simulink model "top_model"  (R2025a)
settings: Solver=ode45  StartTime=0.0  StopTime=2.5  RelTol=1e-3  EnableMultiTasking=on
libraries: spsSeriesRLCBranchLib x3, spsCurrentMeasurementLib x2, spsVoltageMeasurementLib x2, SignalEditorBlockLib x2, spsDiodeLib x1, spsIGBTLib x1, spsPVArrayLib x1, spsPWMGeneratorDCDCLib x1, spsSeriesRLCLoadLib x1, sps_lib x1
settings Model: Creator=The MathWorks, Inc.  LastModifiedBy=Asus
settings SolverCC: AlgebraicLoopSolver=TrustRegion
settings DataIOCC: LimitDataPoints=on  ReturnWorkspaceOutputs=off
settings OptimizationCC: LifeSpan=inf
settings DebuggingCC: UnconnectedInputMsg=warning  UnconnectedOutputMsg=warning  UnconnectedLineMsg=warning  AllowSymbolicDim=off  SFUnexpectedBacktrackingDiag=warning  SFNoUnconditionalDefaultTransitionDiag=warning  SFExecutionAtInitializationDiag=none  ArithmeticOperatorsInVariantConditions=warning
settings ModelReferenceCC: EnableRefExpFcnMdlSchedulingChecks=on  PropagateSignalLabelsOutOfModel=off
settings SFSimCC: SimUseLocalCustomCode=off  CustomCodeUndefinedFunction=UseInterfaceOnly
settings RTWCC: RTWUseLocalCustomCode=off  GPUComputeCapability=3.5
settings CodeAppCC: StateflowObjectComments=on
settings GRTTargetCC: TargetLangStandard=C89/C90 (ANSI)
settings ConfigComp: CovMetricSettings=dw  CovSaveCumulativeToWorkspaceVar=on  CovSaveSingleToWorkspaceVar=on  CovExternalEMLEnable=off

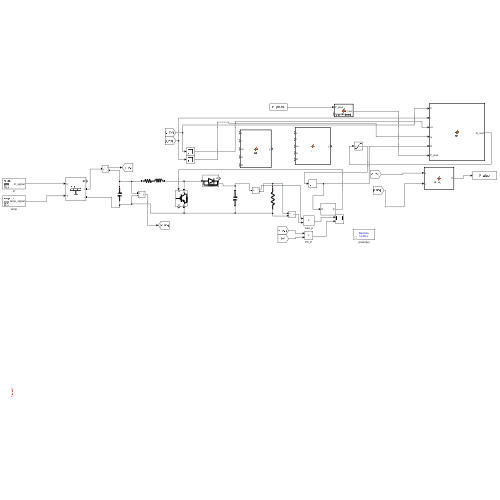
[thumbnail: Simulink's stored preview of the top-level diagram]
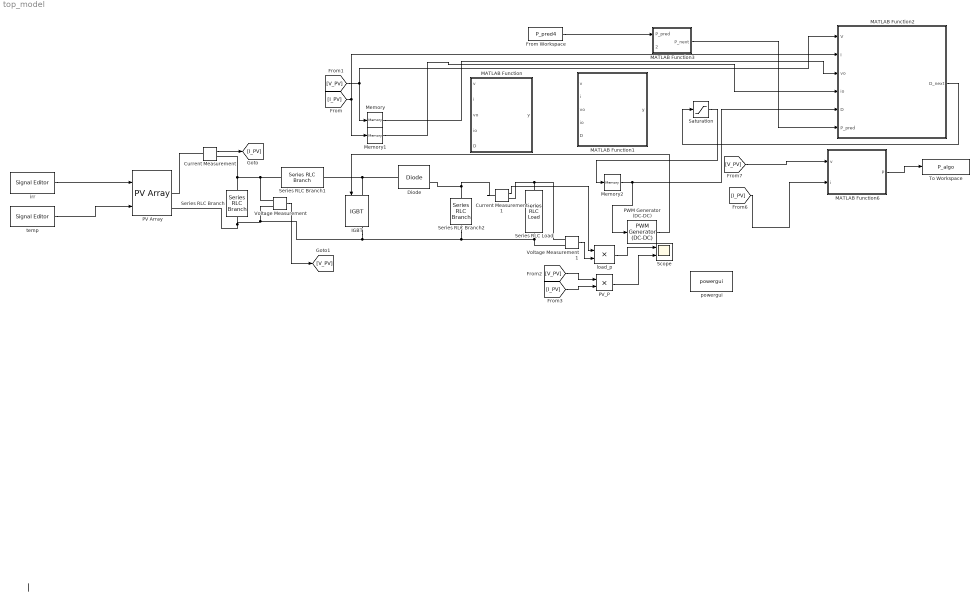
== system top_model ==
  Current Measurement : spsCurrentMeasurementLib/Current Measurement  PhasorSimulation=off  OutputType=Complex  PSBequivalent=0
  Current Measurement1 : spsCurrentMeasurementLib/Current Measurement  PhasorSimulation=off  OutputType=Complex  PSBequivalent=0
  Diode : spsDiodeLib/Diode  Ron=0.001  Lon=0  Vf=0.8  IC=0  UseSnubber=0  Rs=500  Cs=250e-9  Measurements=on
  From Workspace : FromWorkspace  VariableName=P_pred4  SampleTime=0.01
  IGBT : spsIGBTLib/IGBT  Ron=0.001  Lon=0  Vf=1  Tf=1e-6  Tt=2e-6  IC=0  Rs=1e5  Cs=inf  Measurements=on
  MATLAB Function : MATLAB Function  TreatAsAtomicUnit=on
  MATLAB Function1 : MATLAB Function  TreatAsAtomicUnit=on
  MATLAB Function2 : MATLAB Function  TreatAsAtomicUnit=on
  MATLAB Function3 : MATLAB Function  TreatAsAtomicUnit=on
  MATLAB Function6 : MATLAB Function  TreatAsAtomicUnit=on
  Memory : Memory
  Memory1 : Memory
  Memory2 : Memory
  PV Array : spsPVArrayLib/PV Array  Npar=66  Nser=10  PlotType=array @ 1000 W/m2 & specified temperatures  S_vec="[ 1000  500  100 ]"  Temp_C_vec="[ 45 25  ]"  ModuleName=User-defined  PlotWhenSelected=off  Pm=305.226  Ncell=96  Voc=64.2  Isc=5.96  Vm=54.7  Im=5.58  beta_Voc_pc=-0.177  alpha_Isc_pc=0.003516  beta_Voc=-0.11363  alpha_Isc=0.00020955  IL=5.9893  I0=3.2313e-14  nI=0.79323  Rsh=279.5394  Rs=0.53126  RobustModel=off  RobustCellTemperature=313.3991  BAL=on  Tc=1e-6  Tfilter=5e-5
  PV_P : Product
  PWM Generator (DC-DC) : spsPWMGeneratorDCDCLib/PWM Generator (DC-DC)  Fsw=5000  Ts=0
  Saturation : Saturate  UpperLimit=0.9  LowerLimit=0
  Scope : Scope  NumInputPorts=2
      settings: ActiveDisplayYMinimum=-0.098373784311174411  ActiveDisplayYMaximum=0.88536405880057
  Series RLC Branch : spsSeriesRLCBranchLib/Series RLC Branch  LConnTagsString=__new0  RConnTagsString=__new0  BranchType=C  Resistance=1  Inductance=1e-3  SetiL0=off  InitialCurrent=0  Capacitance=100e-6  Setx0=off  InitialVoltage=0  Measurements=None
  Series RLC Branch1 : spsSeriesRLCBranchLib/Series RLC Branch  LConnTagsString=__new0  RConnTagsString=__new0  BranchType=RL  Resistance=0.005  Inductance=0.005  SetiL0=off  InitialCurrent=0  Capacitance=1e-6  Setx0=off  InitialVoltage=0  Measurements=None
  Series RLC Branch2 : spsSeriesRLCBranchLib/Series RLC Branch  LConnTagsString=__new0  RConnTagsString=__new0  BranchType=C  Resistance=1  Inductance=1e-3  SetiL0=off  InitialCurrent=0  Capacitance=12000e-6  Setx0=off  InitialVoltage=0  Measurements=None
  Series RLC Load : spsSeriesRLCLoadLib/Series RLC Load  LConnTagsString=a  RConnTagsString=__new0  NominalVoltage=500  NominalFrequency=50  ActivePower=100e3  InductivePower=0  CapacitivePower=0  Setx0=off  InitialVoltage=0  SetiL0=off  InitialCurrent=0  Measurements=None  LoadType=constant Z
  To Workspace : ToWorkspace  VariableName=P_algo  SaveFormat=Timeseries  SampleTime=-1
  Voltage Measurement : spsVoltageMeasurementLib/Voltage Measurement  PhasorSimulation=off  OutputType=Complex  PSBequivalent=0
  Voltage Measurement1 : spsVoltageMeasurementLib/Voltage Measurement  PhasorSimulation=off  OutputType=Complex  PSBequivalent=0
  irr : SignalEditorBlockLib/Signal Editor  FileName=irr_dataset3.mat  ActiveScenario=irr_ds  ActiveSignal=irr_signal  IsBus=off  OutputBusObjectStr=Bus: BusObject  SampleTime=0.01  ZeroCross=off  OutputAfterFinalValue=Setting to zero  Unit=inherit  PreserveSignalName=on  ApplySigPropsToAllScenarios=off  ApplySigPropsToAllSignals=off  SignalPropertySource=Dialog parameters
  load_p : Product
  powergui : sps_lib/powergui  Priority=1  SimulationMode=Discrete  SampleTime=1e-06  frequency=60  Iterations=50  frequencyindice=0  Pbase=100e6  ErrMax=1e-4  UnitsV=kV  UnitsW=MW  buscounter=0  FunctionMessages=off  echomessages=off  EnableUseOfTLC=off  CurrentSourceSwitches=off  DisableSnubberDevices=off  DisableRonSwitches=off  DisableVfSwitches=off  DisplayEquations=off  AutomaticDiscreteSolvers=off  SolverType=Tustin/Backward Euler (TBE)  Interpol=off  ExternalGateDelay=off  methode=off  Ts=100  x0status=blocks  SPID=on  SwTol=0  HookPort=off  NonlinearTolerance=1e-4  nMaxIteration=100  ContinueOnMaxIteration=off  RestoreLinks=warning  ResistiveCurrentMeasurement=off  Frange=[0:2:500]  Ylog=off  Xlog=on  ShowGrid=off  save=off  variable=ZData  structure=0  ZoomFFT=off  StartTime=0.0  cycles=1  DisplayStyle=1  fundamental=60  FreqAxis=off  MaxFrequency=1000  frequencyindicesteady=1  RmsSteady=1  display=off
  temp : SignalEditorBlockLib/Signal Editor  FileName=temp_dataset3.mat  ActiveScenario=temp_ds  ActiveSignal=temp_signal  IsBus=off  OutputBusObjectStr=Bus: BusObject  SampleTime=0.01  ZeroCross=off  OutputAfterFinalValue=Setting to zero  Unit=inherit  PreserveSignalName=on  ApplySigPropsToAllScenarios=on  ApplySigPropsToAllSignals=off  SignalPropertySource=Dialog parameters
  wires:
  irr/1 -> PV Array/1
  temp/1 -> PV Array/2
  Current Measurement/1 -> [I_PV]
  Voltage Measurement/1 -> [V_PV]
  [V_PV] -> MATLAB Function2/1(V), Memory/1
  [I_PV] -> MATLAB Function2/2(I), Memory1/1
  Saturation/1 -> Memory2/1
  Memory2/1 -> MATLAB Function2/5(D), PWM Generator (DC-DC)/1
  PWM Generator (DC-DC)/1 -> IGBT/1
  Current Measurement1/1 -> load_p/1
  Voltage Measurement1/1 -> load_p/2
  load_p/1 -> Scope/1
  [V_PV] -> PV_P/1
  [I_PV] -> PV_P/2
  PV_P/1 -> Scope/2
  Memory/1 -> MATLAB Function2/3(vo)
  Memory1/1 -> MATLAB Function2/4(io)
  From Workspace/1 -> MATLAB Function3/1(P_pred)
  MATLAB Function3/1(P_next) -> MATLAB Function2/6(P_pred)
  MATLAB Function6/1(P) -> To Workspace/1
  [V_PV] -> MATLAB Function6/1(v)
  [I_PV] -> MATLAB Function6/2(i)
  MATLAB Function2/1(D_next) -> Saturation/1
  connections:
  Current Measurement/LConn1 -- PV Array/RConn1
  Series RLC Branch/RConn1 -- Voltage Measurement1/LConn2 -- Series RLC Load/RConn1 -- Series RLC Branch2/RConn1 -- IGBT/RConn1 -- Voltage Measurement/LConn2 -- PV Array/RConn2
  Voltage Measurement/LConn1 -- Series RLC Branch1/LConn1 -- Series RLC Branch/LConn1 -- Current Measurement/RConn1
  IGBT/LConn1 -- Diode/LConn1 -- Series RLC Branch1/RConn1
  Series RLC Branch2/LConn1 -- Current Measurement1/LConn1 -- Diode/RConn1
  Voltage Measurement1/LConn1 -- Current Measurement1/RConn1 -- Series RLC Load/LConn1
  ?

== matlab function top_model/MATLAB Function1 ==
  data: v input; y output; i input; vo input; io input; D input
function y = po(v, i, vo, io, D)
% MPPT Perturb & Observe (P&O)

d = 5e-5;      % step size
eps = 1e-6;    % small tolerance

% Power
P  = v  * i;
Po = vo * io;

% Delta
dP = P - Po;
dV = v - vo;

m = D;

if abs(dP) < eps
    % Power not change -> keep duty
    m = D;
else
    if dP > 0
        % Power increased
        if dV > 0
            m = D + d;
        else
            m = D - d;
        end
    else
        % Power decreased
        if dV > 0
            m = D - d;
        else
            m = D + d;
        end
    end
end

% Limit duty cycle
m = min(max(m, 0), 1);

y = m;
end

== matlab function top_model/MATLAB Function ==
  data: v input; y output; i input; vo input; io input; D input
function y = inc(v, i, vo, io, D)

d = 5e-5;
eps = 1e-6;

dv = v - vo;
di = i - io;

m = D;

if abs(dv) < eps
    if abs(di) < eps
        m = D;
    elseif di > 0
        m = D - d;
    else
        m = D + d;
    end
else
    if abs(di/dv + i/v) < eps
        m = D;
    elseif di/dv > -i/v
        m = D - d;
    else
        m = D + d;
    end
end

% limit duty cycle
m = min(max(m,0),1);

y = m;
end

== matlab function top_model/MATLAB Function2 ==
  data: V input; D_next output; I input; vo input; io input; D input; P_pred input
function D_next = fcn(V,I,vo,io,D,P_pred)
%#codegen
% AI-MPPT with Temporal Fusion (PAST + FUTURE)
% Codegen & Simulink safe implementation

%% ===== Persistent States =====
persistent init V_f I_f P_hist V_hist ai_conf momentum converge_cnt pred_mom

if isempty(init)
    init = true;
    V_f = V;
    I_f = I;

    P_hist = ones(10,1)*(V*I);
    V_hist = ones(10,1)*V;

    ai_conf = 0.8;
    momentum = 0;
    converge_cnt = 0;
    pred_mom = 0;
end

%% ===== Constants =====
Vmpp_stc = 54.7;
Pmpp_stc = Vmpp_stc*5.58;

D_min = 0.05;
D_max = 0.95;

d_min = 1.5e-4;
d_max = 0.02;

alpha_v = 0.82;
ai_thr  = 0.30;
ai_decay = 0.96;
err_gain = 10;

mom_k = 0.55;
rate_n = 0.05;
rate_f = 0.10;

%% ===== Input Protection =====
if vo == 0, vo = V; end
if io == 0, io = I; end

%% ===== Adaptive Filtering =====
is_tr = (abs(V-vo) > 0.5) || (abs(I-io) > 0.1);
if is_tr
    a = 0.68;
else
    a = alpha_v;
end

V_f = a*V + (1-a)*V_f;
I_f = a*I + (1-a)*I_f;
P_now = V_f*I_f;

%% ===== Update History =====
P_hist(1:end-1) = P_hist(2:end);
P_hist(end) = P_now;

V_hist(1:end-1) = V_hist(2:end);
V_hist(end) = V_f;

P_diff = diff(P_hist);     % 9x1
V_diff = diff(V_hist);     % 9x1

%% ===== PAST: Trend & Gradient =====
weights = [0.03;0.05;0.07;0.10;0.13;0.15;0.17;0.20;0.10];
trend_score = sum(weights .* sign(P_diff));

% Gradient estimation (safe)
sum_g = 0;
cnt_g = 0;
for k = 1:9
    if abs(V_diff(k)) > 1e-3
        sum_g = sum_g + P_diff(k)/V_diff(k);
        cnt_g = cnt_g + 1;
    end
end

if cnt_g > 0
    avg_gradient = sum_g/cnt_g;
    gradient_stable = true;
else
    avg_gradient = 0;
    gradient_stable = false;
end

%% ===== Consistency =====
consistency = 0;
for k = 6:9
    if sign(P_diff(k)) == sign(P_diff(9))
        consistency = consistency + 1;
    end
end
consistency = consistency / 4;

%% ===== FUTURE: AI Prediction =====
P_pred_ok = (P_pred > 1) && (P_pred < 2*Pmpp_stc);

if P_pred_ok
    P_err = (P_pred - P_now)/max(P_pred,1);
    qual = 1 - min(abs(P_err),1);
    ai_conf = 0.35*qual + 0.65*ai_conf;

    pred_dir = sign(P_pred - P_now);
    pred_mom = 0.7*pred_mom + 0.3*pred_dir;

    gain = 0.18 + 0.12*min(abs(P_err),0.6);
    Vmpp_pred = V_f + gain*Vmpp_stc*sign(P_err);
else
    P_err = 0;
    ai_conf = max(ai_conf*ai_decay,0.3);
    Vmpp_pred = V_f;
end

%% ===== FUSION =====
if ai_conf > 0.7 && P_pred_ok
    w_p = 0.3; w_f = 0.7;
elseif ai_conf > 0.5 && P_pred_ok
    w_p = 0.5; w_f = 0.5;
else
    w_p = 0.7; w_f = 0.3;
end

if abs(avg_gradient) > 0.1
    dir_past = sign(avg_gradient);
else
    dir_past = sign(trend_score);
end
if dir_past == 0, dir_past = 1; end

dir_future = sign(Vmpp_pred - V_f);
dir = sign(w_p*dir_past + w_f*dir_future);
if dir == 0, dir = 1; end
if P_pred_ok && abs(P_err) < 0.03
    dir = sign(dir + 0.35*sign(P_pred - P_now));
end
if dir == 0
    dir = 1;
end

%% ===== Convergence =====
near_pred = abs(P_err) < 0.012;
near_grad = gradient_stable && abs(avg_gradient) < 0.5;

if near_pred && near_grad
    converge_cnt = min(converge_cnt+1,20);
else
    converge_cnt = max(converge_cnt-1,0);
end
converged = (converge_cnt > 12) && (abs(avg_gradient) < 0.3);


%% ===== Step Size =====
if ai_conf > ai_thr && P_pred_ok
    mag = min(abs(P_err)*err_gain,1);
    step = d_min + (d_max-d_min)*mag;
else
    step = d_min*2;
end

if consistency > 0.7
    step = step*1.2;
end

step = min(step,d_max);

%% ===== Momentum =====
momentum = mom_k*momentum + (1-mom_k)*step;

if converged
    step_f = max(momentum*0.30, d_min*3);
elseif near_pred
    step_f = momentum*0.45;
else
    step_f = momentum;
end


%% ===== Duty Update =====
D_raw = D + dir*step_f;

Vmpp_hat = w_p*V_f + w_f*Vmpp_pred;
D_phy_max = min(D_max, max(1 - Vmpp_hat/max(V_f,1), D_min));

D_next = min(max(D_raw,D_min),D_phy_max);

%% ===== Rate Limit =====
if converged
    rate = 0.008;
elseif is_tr
    rate = rate_f;
else
    rate = rate_n;
end

dD = D_next - D;
if abs(dD) > rate
    D_next = D + sign(dD)*rate;
end

D_next = min(max(D_next,0),1);

end

== matlab function top_model/MATLAB Function3 ==
  data: P_pred input; P_next output; timestamp input
function P_next = get_P_pred(P_pred, timestamp)
    persistent k
    if timestamp < 0.10
        P_next = 0; % หรือค่าที่เหมาะสม
        return;
    end

    if isempty(k)
        k = 1;
    end

    P_next = P_pred(k);
    k = k + 1;
    if k > length(P_pred)
        k = length(P_pred); % หรือวนกลับ = 1
    end
end

== matlab function top_model/MATLAB Function6 ==
  data: v input; P output; i input
function P = P_algo(v, i)
% v,i เป็นค่าที่เกิดจาก duty cycle ของ algorithm ณ เวลานั้น
P = v .* i;   % instantaneous PV power
end
